simulink model "SET1"  (Simulink 5.0)
settings: Solver=ode45  StartTime=0.0  StopTime=10.0  RelTol=1e-3
settings Model: LastModifiedBy=Administrator

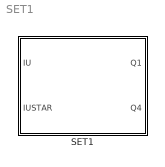
== system SET1 ==
  SET1 : Stateflow chart

== stateflow chart SET1 ==
  settings: updateMethod=CONTINUOUS  executeAtInitialization=1
  state A/
    state A1/
      during:Q1=1;Q4=0;
    state A2/
      during:Q4=1;Q1=0;
    A1 -> A2 : [IU>IUSTAR]
    A2 -> A1 : [IU<IUSTAR]
    (default) -> A1 : [1]
  (default) -> A : [1]
  data: IU input double; IUSTAR input double; Q1 output double; Q4 output double
